simulink model "rtds_opal_aurora_synchronized_2_sc_console"  (Simulink 10.0)
settings: Solver=ode4  StartTime=0.0  StopTime=inf  FixedStep=5e-05  RelTol=1e-3
PreLoadFcn:
  | Ts=50e-6;
InitFcn:
  | Ts=50e-6;
libraries: opal_lib x2
Description:
  | Model of a simple control system for use iin training.
settings Model: Creator=Paul Baracos  LastModifiedBy=nei
settings DataIOCC: LimitDataPoints=on  SignalLoggingSaveFormat=ModelDataLogs  SaveOutput=off  SaveTime=off  SignalLoggingName=sigsOut
settings OptimizationCC: BlockReduction=off  BooleanDataType=off  OptimizeBlockIOStorage=off  BufferReuse=off  GlobalBufferReuse=off  ExpressionFolding=off  LocalBlockOutputs=off  InitFltsAndDblsToZero=on  OptimizeDataStoreBuffers=off  BusAssignmentInplaceUpdate=off
settings DebuggingCC: SaveWithParameterizedLinksMsg=none  SignalResolutionControl=TryResolveAllWithWarning  MultiTaskDSMMsg=warning  MultiTaskCondExecSysMsg=none  FcnCallInpInsideContextMsg=warning
settings HardwareCC: TargetUnknown=on
settings RTWCC: GenCodeOnly=on
settings GRTTargetCC: TargetFcnLib=ansi_tfl_tmw.mat  GeneratePreprocessorConditionals=Disable all
settings ConfigComp: CovExternalEMLEnable=off

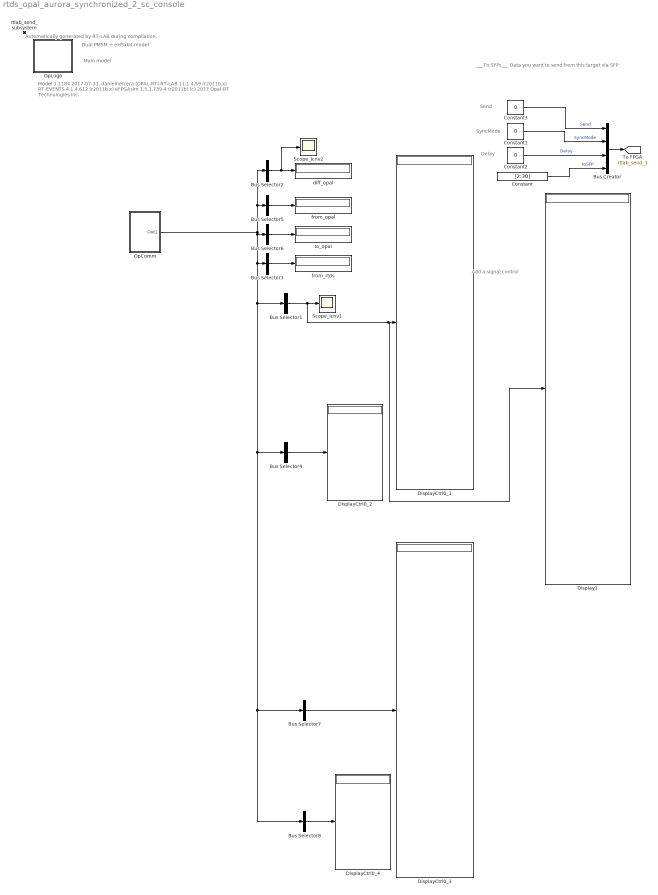
== system rtds_opal_aurora_synchronized_2_sc_console ==
  note: Automatically generated by RT-LAB during compilation.
  note: Model                1.1184         2017-07-31, danielherrera (OPAL-RT)
      | RT-LAB            11.1.4.59    (r2011b.x)
      | RT-EVENTS    4.1.4.612      (r2011b.x)
      | eFPGAsim       1.5.1.739-4  (r2011b)
      | (c) 2017 Opal-RT Technologies Inc.
  note: Main model
  note: Dual PMSM + eHSx64 model
  note: ___To SFPs___
      | Data you want to send from this target via SFP
  note: Add a signal control
  note: SyncMode
  note: Delay
  note: Send
  Bus Creator : BusCreator  Inputs=4
  Bus Selector1 : BusSelector  OutputSignals=SFP_RX_Data (signal 2)  OutputAsBus=on
  Bus Selector2 : BusSelector  OutputSignals=diff_opal (signal 3)  OutputAsBus=on
  Bus Selector3 : BusSelector  OutputSignals=from_rtds (signal 6)  OutputAsBus=on
  Bus Selector4 : BusSelector  OutputSignals=SFP_Status (signal 1)  OutputAsBus=on
  Bus Selector5 : BusSelector  OutputSignals=from_opal (signal 4)  OutputAsBus=on
  Bus Selector6 : BusSelector  OutputSignals=to_opal (signal 5)  OutputAsBus=on
  Bus Selector7 : BusSelector  OutputSignals=SFP_RX_Data (signal 8)  OutputAsBus=on
  Bus Selector8 : BusSelector  OutputSignals=SFP_Status (signal 7)  OutputAsBus=on
  Constant : Constant  Value=[2:30]
  Constant1 : Constant  Value=0  OutDataTypeStr=double
  Constant2 : Constant  Value=0  OutDataTypeStr=double
  Constant3 : Constant  Value=0  OutDataTypeStr=double
  Display1 : Display
  DisplayCtrl0_{1..4} (4 alike) : Display
  OpComm : Subsystem
      mask init:
      | opmaskdisplay('maskdisplay_block',gcb,'disp(''OpComm'')');
      mask Display:
      | patch([0 0.5 0.7 0],[1 1 0 0],[0.7 0.75 0.9]);
      | patch([1 0.53 0.73 1],[1 1 0 0],[1 0.8 0.7]);
      | plot([0 0 1 1 0],[0 1 1 0 0]);
      | disp('OpComm')
  OpLogo : Subsystem
      mask Display:
      | opLogo = imread('efsOpLogo.tif','tif');
      | image(opLogo(:,:,1:3));
  Scope_Icnv1 : Scope
  Scope_Icnv2 : Scope
  diff_opal : Display
  from_opal : Display
  from_rtds : Display
  rtlab_send_subsystem : Subsystem  Priority=-100
      mask Display: text(0,0,'');
  to_opal : Display
  tag scope: rtlab_send_1=global
  wires:
  Bus Selector7/1 -> DisplayCtrl0_3/1
  Bus Selector8/1 -> DisplayCtrl0_4/1
  OpComm/1(Out1) -> Bus Selector5/1, Bus Selector2/1, Bus Selector6/1, Bus Selector8/1, Bus Selector7/1, Bus Selector4/1, Bus Selector1/1, Bus Selector3/1
  Bus Selector6/1 -> to_opal/1
  Bus Selector5/1 -> from_opal/1
  Bus Selector3/1 -> from_rtds/1
  Bus Selector2/1 -> Scope_Icnv2/1, diff_opal/1
  Constant3/1 -> Bus Creator/1  "Send"
  Constant2/1 -> Bus Creator/3  "Delay"
  Constant/1 -> Bus Creator/4  "toSFP"
  Constant1/1 -> Bus Creator/2  "SyncMode"
  Bus Creator/1 -> [rtlab_send_1]
  Bus Selector4/1 -> DisplayCtrl0_2/1
  Bus Selector1/1 -> Display1/1, DisplayCtrl0_1/1, Scope_Icnv1/1

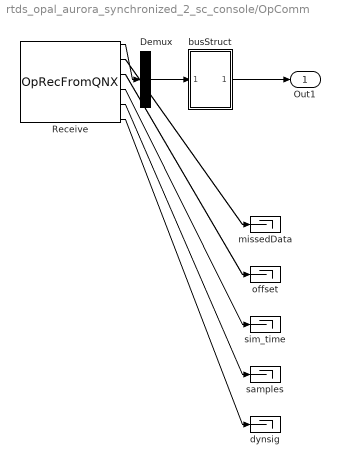
== system rtds_opal_aurora_synchronized_2_sc_console/OpComm ==
  Demux : Demux  Outputs=[78]
  Receive : opal_lib/Communication/OpRecFromQNX  Node_num=1  Acqu_Group=1  Data_Width=78  Synchronization=on  Interpolation=on  Threshold=1.0  modelname=rtds_opal_aurora_synchronized.mdl  sampletime=5e-05
  busStruct : Subsystem
  dynsig : Terminator
  missedData : Terminator
  offset : Terminator
  samples : Terminator
  sim_time : Terminator
  Out1 : Outport
  wires:
  Demux/1 -> busStruct/1(In1)
  busStruct/1(Out1) -> Out1/1
  Receive/1 -> Demux/1
  Receive/6 -> dynsig/1
  Receive/5 -> samples/1
  Receive/4 -> sim_time/1
  Receive/3 -> offset/1
  Receive/2 -> missedData/1

== system rtds_opal_aurora_synchronized_2_sc_console/OpLogo ==

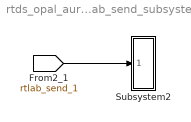
== system rtds_opal_aurora_synchronized_2_sc_console/rtlab_send_subsystem ==
  Subsystem2 : Subsystem
  wires:
  [rtlab_send_1] -> Subsystem2/1(In1)

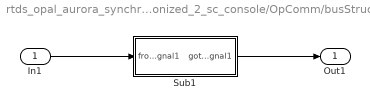
== system rtds_opal_aurora_synchronized_2_sc_console/OpComm/busStruct ==
  In1 : Inport
  Sub1 : Subsystem
  Out1 : Outport
  wires:
  Sub1/1(goto_signal1) -> Out1/1
  In1/1 -> Sub1/1(from_signal1)

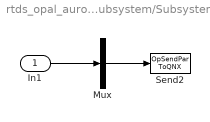
== system rtds_opal_aurora_synchronized_2_sc_console/rtlab_send_subsystem/Subsystem2 ==
  In1 : Inport  PortDimensions=32
  Mux : Mux  Inputs=1
  Send2 : opal_lib/Communication/OpSendPar ToQNX  Node_num=1  modelname=rtds_opal_aurora_synchronized
  wires:
  Mux/1 -> Send2/1
  In1/1 -> Mux/1

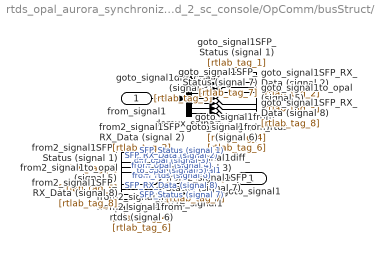
== system rtds_opal_aurora_synchronized_2_sc_console/OpComm/busStruct/Sub1 ==
  from_signal1 : Inport
  buscre_signal1 : BusCreator  Inputs=8
  demux_signal1 : Demux  Outputs="[5  32   1   1   1   1   5  32]"
  goto_signal1 : Outport
  wires:
  buscre_signal1/1 -> goto_signal1/1  "signal1"
  [rtlab_tag_8] -> buscre_signal1/8  "SFP_RX_Data (signal 8)"
  [rtlab_tag_7] -> buscre_signal1/7  "SFP_Status (signal 7)"
  [rtlab_tag_6] -> buscre_signal1/6  "from_rtds (signal 6)"
  [rtlab_tag_5] -> buscre_signal1/5  "to_opal (signal 5)"
  [rtlab_tag_4] -> buscre_signal1/4  "from_opal (signal 4)"
  [rtlab_tag_3] -> buscre_signal1/3  "diff_opal (signal 3)"
  [rtlab_tag_2] -> buscre_signal1/2  "SFP_RX_Data (signal 2)"
  [rtlab_tag_1] -> buscre_signal1/1  "SFP_Status (signal 1)"
  demux_signal1/8 -> [rtlab_tag_8]
  demux_signal1/7 -> [rtlab_tag_7]
  demux_signal1/6 -> [rtlab_tag_6]
  demux_signal1/5 -> [rtlab_tag_5]
  demux_signal1/4 -> [rtlab_tag_4]
  demux_signal1/3 -> [rtlab_tag_3]
  demux_signal1/2 -> [rtlab_tag_2]
  demux_signal1/1 -> [rtlab_tag_1]
  from_signal1/1 -> demux_signal1/1
